simulink model "MesurementUnit"  (R2022a)
settings: Solver=ode23t  StartTime=0.0  StopTime=20  MaxStep=1e-5  RelTol=1e-3  AbsTol=1e-3
libraries: eeGeneralControl x4, SignalEditorBlockLib x1
settings Model: PacingRate=1000  Creator=ykamatan  LastModifiedBy=ykamatan
settings SolverCC: AutoScaleAbsTol=off  SolverJacobianMethodControl=SparsePerturbation  DaesscMode=Fast
settings DataIOCC: SaveOutput=off  SaveTime=off
settings DebuggingCC: UnconnectedInputMsg=warning  UnconnectedOutputMsg=warning  UnconnectedLineMsg=warning  SymbolicDimsDataTypeCodeGenerationDiagnostic=none  SFMachineParentedDataDiag=warning
settings SFSimCC: CustomCodeUndefinedFunction=UseInterfaceOnly
settings RTWCC: DLArmComputeVersion=19.05
settings SimscapeCC: SimscapeLogDataHistory=10000

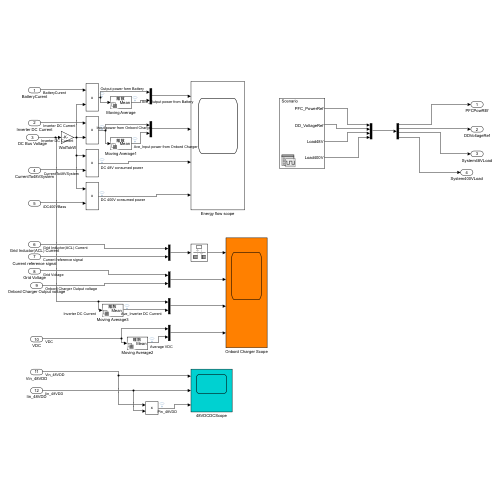
[thumbnail: Simulink's stored preview of the top-level diagram]
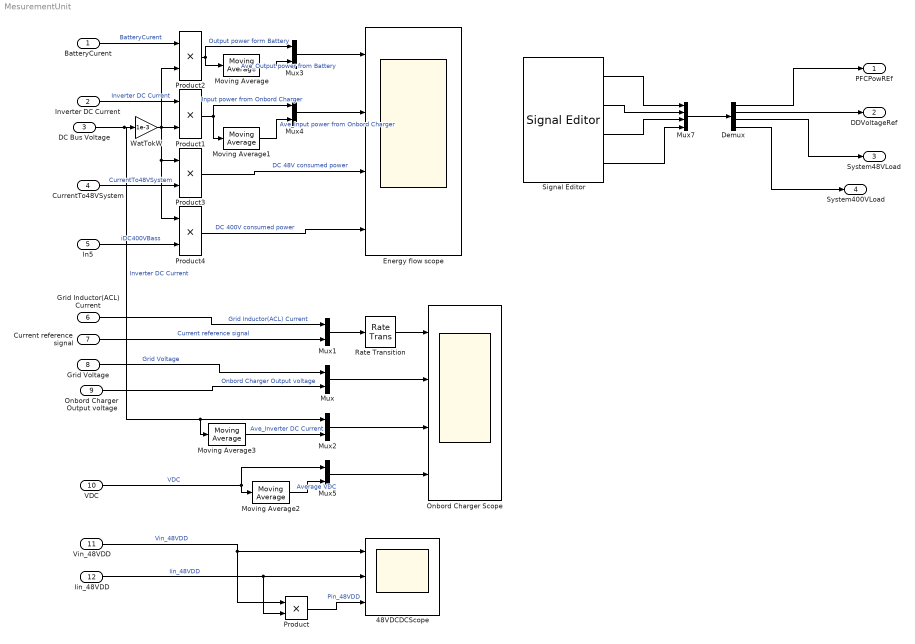
== system MesurementUnit ==
  BatteryCurent : Inport  OutDataTypeStr=double  PortDimensions=1  SampleTime=0
  Inverter DC Current : Inport  Port=2  OutDataTypeStr=double  PortDimensions=1  SampleTime=0
  DC Bus Voltage : Inport  Port=3  OutDataTypeStr=double  PortDimensions=1  SampleTime=0
  CurrentTo48VSystem : Inport  Port=4  OutDataTypeStr=double  PortDimensions=1  SampleTime=0
  In5 : Inport  Port=5  OutDataTypeStr=double  PortDimensions=1  SampleTime=0
  Grid Inductor(ACL) Current : Inport  Port=6  OutDataTypeStr=double  PortDimensions=1  SampleTime=0
  Current reference signal : Inport  Port=7  OutDataTypeStr=double  PortDimensions=1  SampleTime=[0,1]
  Grid Voltage : Inport  Port=8  OutDataTypeStr=double  PortDimensions=1  SampleTime=0
  Onbord Charger Output voltage : Inport  Port=9  OutDataTypeStr=double  PortDimensions=1  SampleTime=0
  VDC : Inport  Port=10  OutDataTypeStr=double  PortDimensions=1  SampleTime=0
  Vin_48VDD : Inport  Port=11  OutDataTypeStr=double  PortDimensions=1  SampleTime=0
  Iin_48VDD : Inport  Port=12  OutDataTypeStr=double  PortDimensions=1  SampleTime=0
  48VDCDCScope : Scope  NumInputPorts=3
  Demux : Demux
  Energy flow scope : Scope  NumInputPorts=4
  Moving Average : eeGeneralControl/Moving Average  VariantControl=Variant1  LabelModeActiveChoice=Discrete  f=120  x0=0  BufferSize=8192  Ts=1/120/2
      settings: SourceProductBaseCode=PS
  Moving Average1 : eeGeneralControl/Moving Average  VariantControl=Variant1  LabelModeActiveChoice=Discrete  f=120  x0=0  BufferSize=8192  Ts=1/120/2
      settings: SourceProductBaseCode=PS
  Moving Average2 : eeGeneralControl/Moving Average  VariantControl=Variant1  LabelModeActiveChoice=Discrete  f=120  x0=400  BufferSize=8192  Ts=1/120/2
      settings: SourceProductBaseCode=PS
  Moving Average3 : eeGeneralControl/Moving Average  VariantControl=Variant1  LabelModeActiveChoice=Discrete  f=120  x0=0  BufferSize=8192  Ts=1/120/2
      settings: SourceProductBaseCode=PS
  Mux{,1..5} (6 alike) : Mux  Inputs=2
  Mux7 : Mux
  Onbord Charger Scope : Scope  NumInputPorts=4
  Product{,1..4} (5 alike) : Product
  Rate Transition : RateTransition
  Signal Editor : SignalEditorBlockLib/Signal Editor  FileName=InputSignal.mat  ActiveScenario=Scenario  ActiveSignal=PFC_PowerRef  IsBus=off  OutputBusObjectStr=Bus: BusObject  SampleTime=-1  ZeroCross=off  OutputAfterFinalValue=Setting to zero  Unit=inherit  PreserveSignalName=on
  WatTokW : Gain  Gain=1e-3
  PFCPowREf : Outport  OutDataTypeStr=double  PortDimensions=1  SampleTime=0
  DDVoltageRef : Outport  Port=2  OutDataTypeStr=double  PortDimensions=1  SampleTime=0
  System48VLoad : Outport  Port=3
  System400VLoad : Outport  Port=4
  wires:
  Product1/1 -> Moving Average1/1, Mux4/1  "Input power from Onbord Charger"
  Iin_48VDD/1 -> 48VDCDCScope/2, Product/2  "Iin_48VDD"
  Mux/1 -> Onbord Charger Scope/2
  Moving Average/1 -> Mux3/2  "Ave_Output power from Battery"
  Vin_48VDD/1 -> 48VDCDCScope/1, Product/1  "Vin_48VDD"
  Product/1 -> 48VDCDCScope/3  "Pin_48VDD"
  WatTokW/1 -> Product4/1, Product3/1, Product1/2, Product2/2
  Mux2/1 -> Onbord Charger Scope/3
  Product4/1 -> Energy flow scope/4  "DC 400V consumed power"
  DC Bus Voltage/1 -> Moving Average3/1, Mux2/1, WatTokW/1  "Inverter DC Current"
  Mux1/1 -> Rate Transition/1
  Product3/1 -> Energy flow scope/3  "DC 48V consumed power"
  Mux3/1 -> Energy flow scope/1
  Moving Average1/1 -> Mux4/2  "Ave_Input power from Onbord Charger"
  Moving Average3/1 -> Mux2/2  "Ave_Inverter DC Current"
  Onbord Charger Output voltage/1 -> Mux/2  "Onbord Charger Output voltage"
  VDC/1 -> Mux5/1, Moving Average2/1  "VDC"
  Mux5/1 -> Onbord Charger Scope/4
  Mux4/1 -> Energy flow scope/2
  Grid Inductor(ACL) Current/1 -> Mux1/1  "Grid Inductor(ACL) Current"
  Moving Average2/1 -> Mux5/2  "Average VDC"
  Product2/1 -> Moving Average/1, Mux3/1  "Output power form Battery"
  Current reference signal/1 -> Mux1/2  "Current reference signal"
  Grid Voltage/1 -> Mux/1  "Grid Voltage"
  BatteryCurent/1 -> Product2/1  "BatteryCurent"
  CurrentTo48VSystem/1 -> Product3/2  "CurrentTo48VSystem"
  Inverter DC Current/1 -> Product1/1  "Inverter DC Current"
  In5/1 -> Product4/2  "iDC400VBass"
  Mux7/1 -> Demux/1
  Demux/1 -> PFCPowREf/1
  Demux/2 -> DDVoltageRef/1
  Demux/3 -> System48VLoad/1
  Demux/4 -> System400VLoad/1
  Signal Editor/1 -> Mux7/1
  Signal Editor/3 -> Mux7/3
  Signal Editor/2 -> Mux7/2
  Signal Editor/4 -> Mux7/4
  Rate Transition/1 -> Onbord Charger Scope/1
